simulink model "ME575ControlAnalysis2sim"  (R2019b)
settings: Solver=ode8  StartTime=Tstart  StopTime=Tend  FixedStep=Tstep  RelTol=1e-3
values from neighbouring files (symbols this model uses):
  denC = [1 0]    [ME575ControlAnalysis2.m]    (also in Update 10.m; Update 9.m; full_proj_script.m)
  denDeltaA = [0.01 1]    [ME575ControlAnalysis2.m]    (also in Update 10.m; Update 9.m; full_proj_script.m)
  denDeltaM = [1 20 100]    [ME575ControlAnalysis2.m]    (also in Update 10.m; Update 9.m; full_proj_script.m)
  denP = [1 0 0]    [ME575ControlAnalysis2.m]    (also in Update 10.m = [0.01736 62 2500 0.7]; Update 9.m = [0.01736 62 146515.68 2064.446]; full_proj_script.m = [0.01736 62 2500 0.7])
  numC = [Kgain Kgain]    [ME575ControlAnalysis2.m]    (also in Update 10.m; Update 9.m; full_proj_script.m)
  numDeltaA = [0.001]    [ME575ControlAnalysis2.m]    (also in Update 10.m; Update 9.m; full_proj_script.m)
  numDeltaM = [0]    [ME575ControlAnalysis2.m]    (also in Update 10.m; Update 9.m; full_proj_script.m)
  numP = [2.236, 6.63e-14]    [ME575ControlAnalysis2.m]    (also in Update 10.m = [608.2]; Update 9.m = [144015.678 2063.744]; full_proj_script.m = [608.2])
settings Model: Creator=Kartik Ariyur  LastModifiedBy=Kartik Ariyur

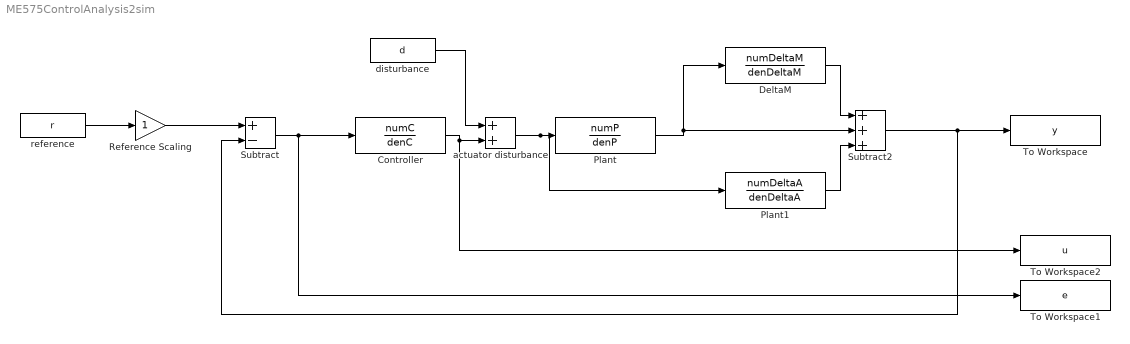
== system ME575ControlAnalysis2sim ==
  Controller : TransferFcn  Numerator=numC  Denominator=denC
  DeltaM : TransferFcn  Numerator=numDeltaM  Denominator=denDeltaM
  Plant : TransferFcn  Numerator=numP  Denominator=denP
  Plant1 : TransferFcn  Numerator=numDeltaA  Denominator=denDeltaA
  Reference Scaling : Gain
  Subtract : Sum  Inputs=+-
  Subtract2 : Sum  Inputs=+++
  To Workspace : ToWorkspace  VariableName=y  SaveFormat=Timeseries  SampleTime=-1
  To Workspace1 : ToWorkspace  VariableName=e  SaveFormat=Timeseries  SampleTime=-1
  To Workspace2 : ToWorkspace  VariableName=u  SaveFormat=Timeseries  SampleTime=-1
  actuator disturbance : Sum
  disturbance : FromWorkspace  VariableName=d  SampleTime=0
  reference : FromWorkspace  VariableName=r  SampleTime=0
  wires:
  Controller/1 -> To Workspace2/1, actuator disturbance/2
  Plant/1 -> DeltaM/1, Subtract2/2
  Subtract/1 -> To Workspace1/1, Controller/1
  actuator disturbance/1 -> Plant1/1, Plant/1
  reference/1 -> Reference Scaling/1
  disturbance/1 -> actuator disturbance/1
  Subtract2/1 -> To Workspace/1, Subtract/2
  DeltaM/1 -> Subtract2/1
  Reference Scaling/1 -> Subtract/1
  Plant1/1 -> Subtract2/3
